simulink model "s1_8"  (R2020b)
settings: Solver=VariableStepAuto  StartTime=0.0  StopTime=20  RelTol=1e-3
libraries: simulink x1
settings Model: Creator=huang  LastModifiedBy=huang

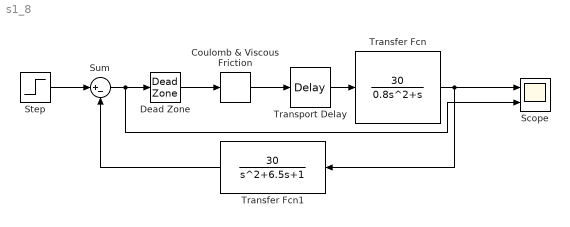
== system s1_8 ==
  Coulomb & Viscous Friction : simulink/Discontinuities/Coulomb & Viscous Friction  offset=2.5  gain=0
  Dead Zone : DeadZone  SaturateOnIntegerOverflow=on
  Scope : Scope  NumInputPorts=2
  Step : Step  Time=0  SampleTime=0
  Sum : Sum  Inputs=|+-
  Transfer Fcn : TransferFcn  Numerator=[30]  Denominator=[0.8 1 0]
  Transfer Fcn1 : TransferFcn  Numerator=[30]  Denominator=[1 6.5 1]
  Transport Delay : TransportDelay  DelayTime=0.4
  wires:
  Dead Zone/1 -> Coulomb & Viscous Friction/1
  Coulomb & Viscous Friction/1 -> Transport Delay/1
  Transport Delay/1 -> Transfer Fcn/1
  Transfer Fcn/1 -> Scope/1, Transfer Fcn1/1
  Sum/1 -> Scope/2, Dead Zone/1
  Transfer Fcn1/1 -> Sum/2
  Step/1 -> Sum/1
